simulink model "phase_jump_a_b_a_2_sc_meter"  (Simulink 9.2)
settings: Solver=ode4  StartTime=0.0  StopTime=101.5  FixedStep=4e-05  RelTol=1e-3
PreLoadFcn:
  | Ts=40e-6;Core_Num = 0;
PostLoadFcn:
  | Ts=40e-6;Core_Num = 0;
InitFcn:
  | Ts=40e-6;Core_Num = 0;
libraries: opal_lib x1
settings Model: ARTEMISmethode_block_infos=$$__separator__$$  Creator=DETLDAQ  LastModifiedBy=DETLDAQ
settings OptimizationCC: BlockReduction=off  BooleanDataType=off  OptimizeBlockIOStorage=off  BufferReuse=off  GlobalBufferReuse=off  ExpressionFolding=off  LocalBlockOutputs=off  OptimizeDataStoreBuffers=off  BusAssignmentInplaceUpdate=off
settings DebuggingCC: SaveWithParameterizedLinksMsg=none  SignalResolutionControl=TryResolveAllWithWarning  MultiTaskDSMMsg=warning  MultiTaskCondExecSysMsg=none  FcnCallInpInsideContextMsg=error
settings HardwareCC: TargetUnknown=on
settings RTWCC: GenCodeOnly=on
settings GRTTargetCC: CombineOutputUpdateFcns=on  GRTInterface=off
settings SimscapeCC: SimscapeNormalizeSystem=off

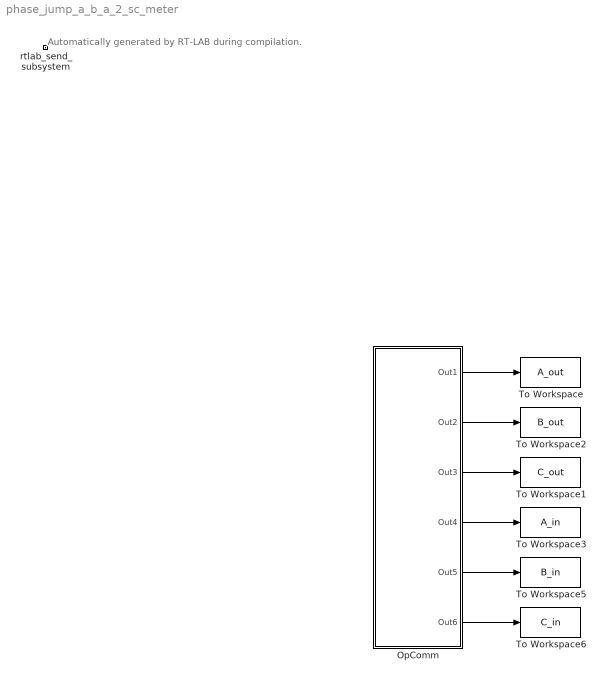
== system phase_jump_a_b_a_2_sc_meter ==
  note: Automatically generated by RT-LAB during compilation.
  OpComm : Subsystem
      mask init:
      | opmaskdisplay('maskdisplay_block',gcb,'disp(''OpComm'')');
      mask Display:
      | patch([0 0.5 0.7 0],[1 1 0 0],[0.7 0.75 0.9]);
      | patch([1 0.53 0.73 1],[1 1 0 0],[1 0.8 0.7]);
      | plot([0 0 1 1 0],[0 1 1 0 0]);
      | disp('OpComm')
  To Workspace : ToWorkspace  VariableName=A_out  SaveFormat=Timeseries  SampleTime=Ts
  To Workspace1 : ToWorkspace  VariableName=C_out  SaveFormat=Timeseries  SampleTime=Ts
  To Workspace2 : ToWorkspace  VariableName=B_out  SaveFormat=Timeseries  SampleTime=Ts
  To Workspace3 : ToWorkspace  VariableName=A_in  SaveFormat=Timeseries  SampleTime=Ts
  To Workspace5 : ToWorkspace  VariableName=B_in  SaveFormat=Timeseries  SampleTime=Ts
  To Workspace6 : ToWorkspace  VariableName=C_in  SaveFormat=Timeseries  SampleTime=Ts
  rtlab_send_subsystem : Subsystem  Priority=-100
      mask Display: text(0,0,'');
  wires:
  OpComm/6(Out6) -> To Workspace6/1
  OpComm/5(Out5) -> To Workspace5/1
  OpComm/4(Out4) -> To Workspace3/1
  OpComm/2(Out2) -> To Workspace2/1
  OpComm/3(Out3) -> To Workspace1/1
  OpComm/1(Out1) -> To Workspace/1

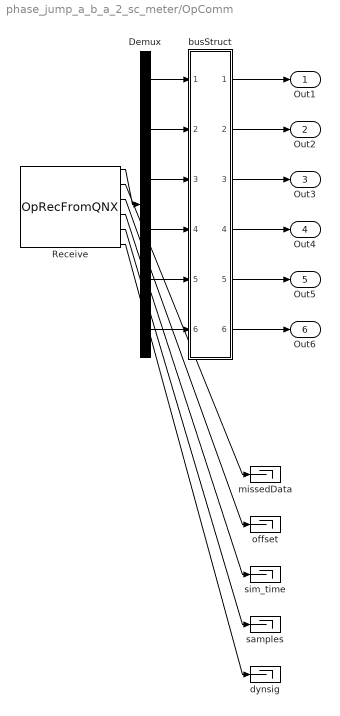
== system phase_jump_a_b_a_2_sc_meter/OpComm ==
  Demux : Demux  Outputs="[1  1  1  1  1  1]"
  Receive : opal_lib/Communication/OpRecFromQNX  Node_num=1  Acqu_Group=1  Data_Width=6  Synchronization=on  Interpolation=on  Threshold=1.0  modelname=Phase_Jump_A_B_A.mdl  sampletime=4e-05
  busStruct : Subsystem
  dynsig : Terminator
  missedData : Terminator
  offset : Terminator
  samples : Terminator
  sim_time : Terminator
  Out1 : Outport
  Out2 : Outport  Port=2
  Out3 : Outport  Port=3
  Out4 : Outport  Port=4
  Out5 : Outport  Port=5
  Out6 : Outport  Port=6
  wires:
  Demux/6 -> busStruct/6(In6)
  Demux/5 -> busStruct/5(In5)
  Demux/4 -> busStruct/4(In4)
  Demux/3 -> busStruct/3(In3)
  Demux/2 -> busStruct/2(In2)
  Demux/1 -> busStruct/1(In1)
  busStruct/6(Out6) -> Out6/1
  busStruct/5(Out5) -> Out5/1
  busStruct/4(Out4) -> Out4/1
  busStruct/3(Out3) -> Out3/1
  busStruct/2(Out2) -> Out2/1
  busStruct/1(Out1) -> Out1/1
  Receive/1 -> Demux/1
  Receive/6 -> dynsig/1
  Receive/5 -> samples/1
  Receive/4 -> sim_time/1
  Receive/3 -> offset/1
  Receive/2 -> missedData/1

== system phase_jump_a_b_a_2_sc_meter/rtlab_send_subsystem ==

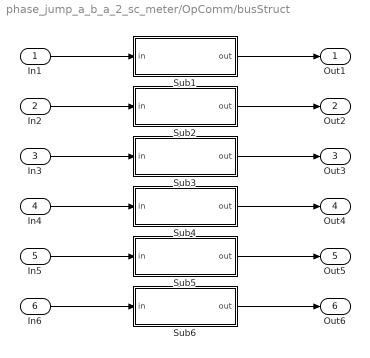
== system phase_jump_a_b_a_2_sc_meter/OpComm/busStruct ==
  In1 : Inport
  In2 : Inport  Port=2
  In3 : Inport  Port=3
  In4 : Inport  Port=4
  In5 : Inport  Port=5
  In6 : Inport  Port=6
  Sub1 : Subsystem
  Sub2 : Subsystem
  Sub3 : Subsystem
  Sub4 : Subsystem
  Sub5 : Subsystem
  Sub6 : Subsystem
  Out1 : Outport
  Out2 : Outport  Port=2
  Out3 : Outport  Port=3
  Out4 : Outport  Port=4
  Out5 : Outport  Port=5
  Out6 : Outport  Port=6
  wires:
  Sub6/1(out) -> Out6/1
  In6/1 -> Sub6/1(in)
  Sub5/1(out) -> Out5/1
  In5/1 -> Sub5/1(in)
  Sub4/1(out) -> Out4/1
  In4/1 -> Sub4/1(in)
  Sub3/1(out) -> Out3/1
  In3/1 -> Sub3/1(in)
  Sub2/1(out) -> Out2/1
  In2/1 -> Sub2/1(in)
  Sub1/1(out) -> Out1/1
  In1/1 -> Sub1/1(in)

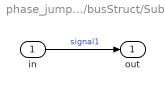
== system phase_jump_a_b_a_2_sc_meter/OpComm/busStruct/Sub1 ==
  in : Inport
  out : Outport
  wires:
  in/1 -> out/1  "signal1"

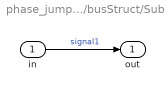
== system phase_jump_a_b_a_2_sc_meter/OpComm/busStruct/Sub2 ==
  in : Inport
  out : Outport
  wires:
  in/1 -> out/1  "signal1"

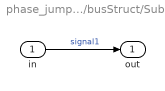
== system phase_jump_a_b_a_2_sc_meter/OpComm/busStruct/Sub3 ==
  in : Inport
  out : Outport
  wires:
  in/1 -> out/1  "signal1"

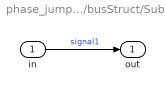
== system phase_jump_a_b_a_2_sc_meter/OpComm/busStruct/Sub4 ==
  in : Inport
  out : Outport
  wires:
  in/1 -> out/1  "signal1"

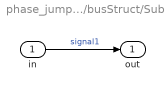
== system phase_jump_a_b_a_2_sc_meter/OpComm/busStruct/Sub5 ==
  in : Inport
  out : Outport
  wires:
  in/1 -> out/1  "signal1"

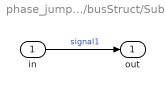
== system phase_jump_a_b_a_2_sc_meter/OpComm/busStruct/Sub6 ==
  in : Inport
  out : Outport
  wires:
  in/1 -> out/1  "signal1"
